simulink model "DC_Electric_Motor"  (R2016b)
settings: Solver=VariableStepAuto  StartTime=0.0  StopTime=3  RelTol=1e-3
values from neighbouring files (symbols this model uses):
  b = 3.5077E-6    (= 3.5077e-06)    [DC_Motor.m]
  J = 3.2284E-6    (= 3.2284e-06)    [DC_Motor.m]
  Kb = 0.0274    [DC_Motor.m]
  Kt = 0.0274    [DC_Motor.m]
  L = 2.75E-6    (= 2.75e-06)    [DC_Motor.m]
  R = 4    [DC_Motor.m]
libraries: simulink x1
settings Model: Creator=1026691  LastModifiedBy=1026691

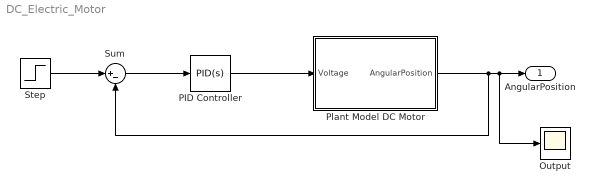
== system DC_Electric_Motor ==
  Output : Scope
  PID Controller : simulink/Continuous/PID Controller  Controller=PID  TimeDomain=Continuous-time  SampleTime=-1  IntegratorMethod=Forward Euler  FilterMethod=Forward Euler  Form=Parallel  UseFilter=on  ControllerParametersSource=internal  P=1  I=1  D=0  N=100  InitialConditionSource=internal  InitialConditionForIntegrator=0  InitialConditionForFilter=0  ExternalReset=none  LimitOutput=off  UpperSaturationLimit=inf  LowerSaturationLimit=-inf  LinearizeAsGain=on  AntiWindupMode=none  Kb=1  TrackingMode=off  Kt=1  PParamMin=[]  PParamMax=[]  IParamMin=[]  IParamMax=[]  DParamMin=[]  DParamMax=[]  NParamMin=[]  NParamMax=[]  KbParamMin=[]  KbParamMax=[]  KtParamMin=[]  KtParamMax=[]  POutMin=[]  POutMax=[]  IOutMin=[]  IOutMax=[]  DOutMin=[]  DOutMax=[]  NOutMin=[]  NOutMax=[]  KbOutMin=[]  KbOutMax=[]  KtOutMin=[]  KtOutMax=[]  IntegratorOutMin=[]  IntegratorOutMax=[]  FilterOutMin=[]  FilterOutMax=[]  SumOutMin=[]  SumOutMax=[]  SumI1OutMin=[]  SumI1OutMax=[]  SumI2OutMin=[]  SumI2OutMax=[]  SumI3OutMin=[]  SumI3OutMax=[]  SumDOutMin=[]  SumDOutMax=[]  SaturationOutMin=[]  SaturationOutMax=[]  IntegratorContinuousStateAttributes=''  IntegratorStateMustResolveToSignalObject=off  IntegratorRTWStateStorageClass=Auto  FilterContinuousStateAttributes=''  FilterStateMustResolveToSignalObject=off  FilterRTWStateStorageClass=Auto  DifferentiatorICPrevScaledInput=0  DifferentiatorOutMin=[]  DifferentiatorOutMax=[]
  Plant Model DC Motor : Subsystem
  Step : Step  SampleTime=0
  Sum : Sum  Inputs=|+-
  AngularPosition : Outport
  wires:
  Plant Model DC Motor/1(AngularPosition) -> Sum/2, Output/1, AngularPosition/1
  PID Controller/1 -> Plant Model DC Motor/1(Voltage)
  Sum/1 -> PID Controller/1
  Step/1 -> Sum/1

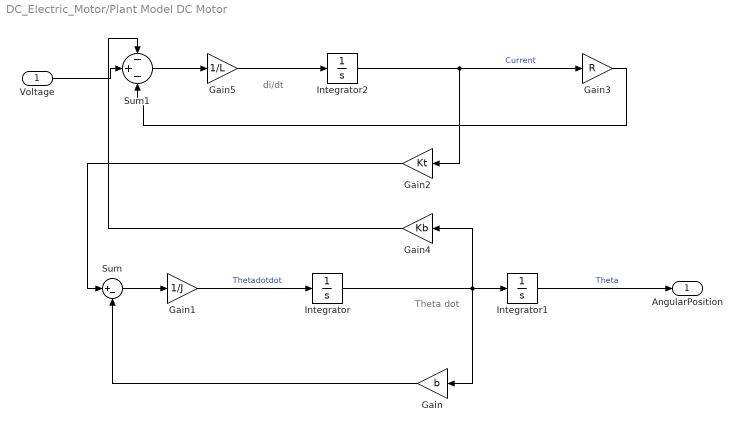
== system DC_Electric_Motor/Plant Model DC Motor ==
  note: di/dt
  note: Theta dot
  Voltage : Inport
  Gain : Gain  Gain=b
  Gain1 : Gain  Gain=1/J
  Gain2 : Gain  Gain=Kt
  Gain3 : Gain  Gain=R
  Gain4 : Gain  Gain=Kb
  Gain5 : Gain  Gain=1/L
  Integrator : Integrator
  Integrator1 : Integrator
  Integrator2 : Integrator
  Sum : Sum  Inputs=|+-
  Sum1 : Sum  Inputs=-+-
  AngularPosition : Outport
  wires:
  Gain4/1 -> Sum1/1
  Sum/1 -> Gain1/1
  Gain2/1 -> Sum/1
  Gain1/1 -> Integrator/1  "Thetadotdot"
  Integrator/1 -> Gain4/1, Gain/1, Integrator1/1
  Integrator1/1 -> AngularPosition/1  "Theta"
  Voltage/1 -> Sum1/2
  Sum1/1 -> Gain5/1
  Gain3/1 -> Sum1/3
  Gain/1 -> Sum/2
  Integrator2/1 -> Gain2/1, Gain3/1  "Current"
  Gain5/1 -> Integrator2/1
